simulink model "test_gain2020a"  (R2020a)
settings: Solver=FixedStepAuto  StartTime=0.0  StopTime=tend  FixedStep=tsamp  RelTol=1e-3
settings Model: Creator=20191777  LastModifiedBy=20191777
settings DebuggingCC: SFMachineParentedDataDiag=error

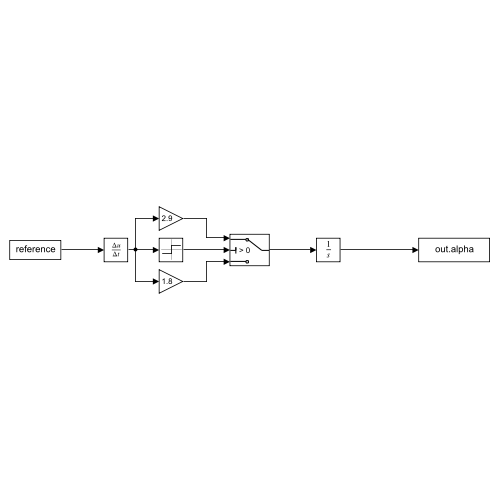
[thumbnail: Simulink's stored preview of the top-level diagram]
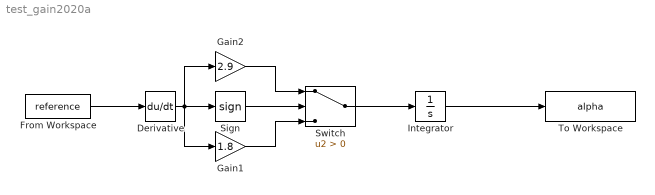
== system test_gain2020a ==
  Derivative : Derivative
  From Workspace : FromWorkspace  VariableName=reference
  Gain1 : Gain  Gain=1.8
  Gain2 : Gain  Gain=2.9
  Integrator : Integrator
  Sign : Signum
  Switch : Switch  Criteria=u2 > Threshold
  To Workspace : ToWorkspace  VariableName=alpha  SaveFormat=Timeseries  SampleTime=-1
  wires:
  From Workspace/1 -> Derivative/1
  Sign/1 -> Switch/2
  Derivative/1 -> Gain1/1, Gain2/1, Sign/1
  Gain2/1 -> Switch/1
  Gain1/1 -> Switch/3
  Switch/1 -> Integrator/1
  Integrator/1 -> To Workspace/1
